simulink model "ESTS_FRIC_HILO_LIM_test"  (R2024b)
settings: Solver=VariableStepAuto  StartTime=0.0  StopTime=10.0  RelTol=1e-3
libraries: ESTS_FRIC_HILO_LIM x1
settings Model: Creator=blatak  LastModifiedBy=blatak

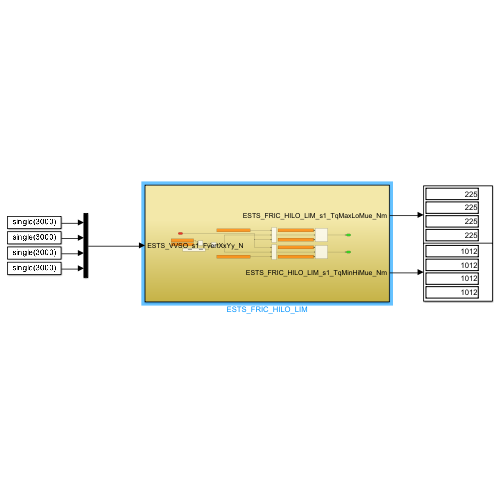
[thumbnail: Simulink's stored preview of the top-level diagram]
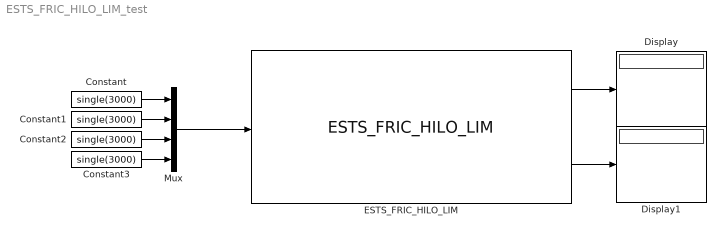
== system ESTS_FRIC_HILO_LIM_test ==
  Constant{,1..3} (4 alike) : Constant  Value=single(3000)
  Display : Display
  Display1 : Display
  ESTS_FRIC_HILO_LIM : ESTS_FRIC_HILO_LIM/ESTS_FRIC_HILO_LIM  SystemSampleTime=-1  VariantActivationTime=update diagram  AllowFlexibleInterface=on  Latency=0  AutoFrameSizeCalculation=off
  Mux : Mux
  wires:
  Constant/1 -> Mux/1
  Constant1/1 -> Mux/2
  Constant2/1 -> Mux/3
  Constant3/1 -> Mux/4
  Mux/1 -> ESTS_FRIC_HILO_LIM/1
  ESTS_FRIC_HILO_LIM/1 -> Display/1
  ESTS_FRIC_HILO_LIM/2 -> Display1/1
